simulink model "mSimpleSubsystemConfig"  (R2019b)
settings: Solver=VariableStepAuto  StartTime=0.0  StopTime=10.0  RelTol=1e-3
libraries: autolibsharedmappedengines x1
(part 1 of 2)
settings Model: Creator=9bt  LastModifiedBy=4qz

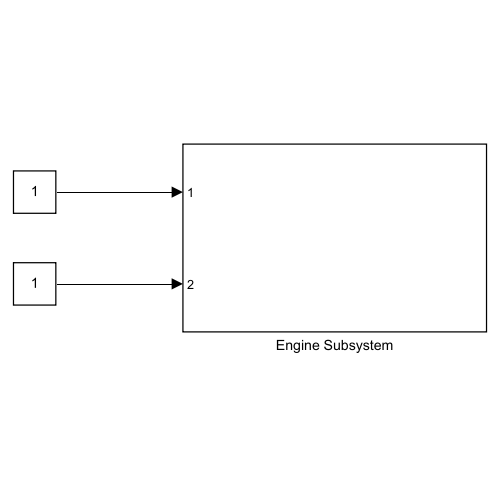
[thumbnail: Simulink's stored preview of the top-level diagram]
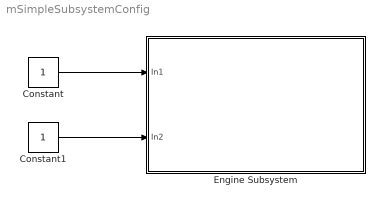
== system mSimpleSubsystemConfig ==
  Constant : Constant
  Constant1 : Constant
  Engine Subsystem : Subsystem
  wires:
  Constant/1 -> Engine Subsystem/1(In1)
  Constant1/1 -> Engine Subsystem/2(In2)
